simulink model "Time_10div"  (R2018a)
settings: Solver=VariableStepAuto  StartTime=0.0  StopTime=40  RelTol=1e-3
libraries: simulink_extras x8
settings Model: Creator=Liuinuy  LastModifiedBy=Liuinuy
settings OptimizationCC: BooleanDataType=off

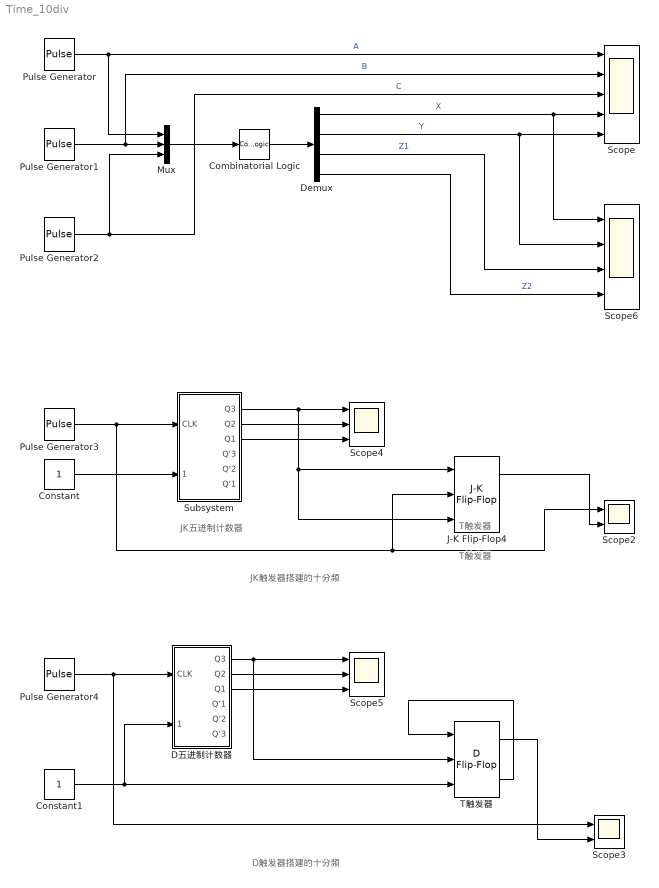
== system Time_10div ==
  note: T触发器
  note: JK触发器搭建的十分频
  note: D触发器搭建的十分频
  note: JK五进制计数器
  note: T触发器
  Combinatorial Logic : CombinatorialLogic  TruthTable=[1 1 1 1;1 0 1 0;1 0 1 0;1 0 1 0;1 0 1 0;1 0 1 0;1 0 1 0;0 1 1 0]
  Constant : Constant  OutDataTypeStr=boolean
  Constant1 : Constant  OutDataTypeStr=boolean
  Demux : Demux
  D五进制计数器 : Subsystem
  J-K Flip-Flop4 : simulink_extras/Flip Flops/J-K Flip-Flop  initial_condition=0
      settings: SourceProductName=Simulink
  Mux : Mux  Inputs=3
  Pulse Generator : DiscretePulseGenerator  Period=8  PulseWidth=4  PhaseDelay=4
  Pulse Generator1 : DiscretePulseGenerator  Period=4  PulseWidth=2  PhaseDelay=2
  Pulse Generator2 : DiscretePulseGenerator  PhaseDelay=1
  Pulse Generator3 : DiscretePulseGenerator
  Pulse Generator4 : DiscretePulseGenerator
  Scope : Scope  NumInputPorts=5
  Scope2 : Scope  NumInputPorts=2
  Scope3 : Scope  NumInputPorts=2
  Scope4 : Scope  NumInputPorts=3
  Scope5 : Scope  NumInputPorts=3
  Scope6 : Scope  NumInputPorts=4
  Subsystem : Subsystem
  T触发器 : simulink_extras/Flip Flops/D Flip-Flop
      settings: SourceProductName=Simulink
  wires:
  Pulse Generator/1 -> Mux/1, Scope/1  "A"
  Pulse Generator1/1 -> Scope/2, Mux/2  "B"
  Pulse Generator2/1 -> Mux/3, Scope/3  "C"
  Mux/1 -> Combinatorial Logic/1
  Combinatorial Logic/1 -> Demux/1
  Demux/1 -> Scope6/1, Scope/4  "X"
  Demux/2 -> Scope6/2, Scope/5  "Y"
  Demux/3 -> Scope6/3  "Z1"
  Demux/4 -> Scope6/4  "Z2"
  J-K Flip-Flop4/1 -> Scope2/2
  Pulse Generator4/1 -> Scope3/1, D五进制计数器/1(CLK)
  Constant1/1 -> D五进制计数器/2(1), T触发器/3
  T触发器/2 -> T触发器/1
  T触发器/1 -> Scope3/2
  Pulse Generator3/1 -> Subsystem/1(CLK), Scope2/1, J-K Flip-Flop4/2
  Subsystem/1(Q3) -> J-K Flip-Flop4/3, J-K Flip-Flop4/1, Scope4/1
  Constant/1 -> Subsystem/2(1)
  D五进制计数器/1(Q3) -> T触发器/2, Scope5/1
  D五进制计数器/3(Q1) -> Scope5/3
  D五进制计数器/2(Q2) -> Scope5/2
  Subsystem/2(Q2) -> Scope4/2
  Subsystem/3(Q1) -> Scope4/3

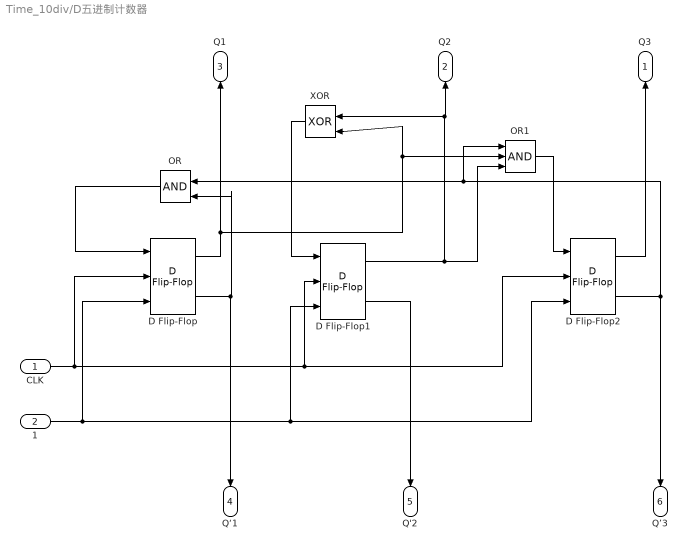
== system Time_10div/D五进制计数器 ==
  CLK : Inport
  1 : Inport  Port=2
  D Flip-Flop : simulink_extras/Flip Flops/D Flip-Flop
      settings: SourceProductName=Simulink
  D Flip-Flop1 : simulink_extras/Flip Flops/D Flip-Flop
      settings: SourceProductName=Simulink
  D Flip-Flop2 : simulink_extras/Flip Flops/D Flip-Flop
      settings: SourceProductName=Simulink
  OR : Logic  IconShape=distinctive  AllPortsSameDT=off  OutDataTypeStr=boolean
  OR1 : Logic  Inputs=3  IconShape=distinctive  AllPortsSameDT=off  OutDataTypeStr=boolean
  XOR : Logic  Operator=XOR  IconShape=distinctive  AllPortsSameDT=off  OutDataTypeStr=boolean
  Q3 : Outport
  Q2 : Outport  Port=2
  Q1 : Outport  Port=3
  Q‘1 : Outport  Port=4
  Q'2 : Outport  Port=5
  Q’3 : Outport  Port=6
  wires:
  D Flip-Flop/1 -> Q1/1, OR1/2, XOR/2
  OR/1 -> D Flip-Flop/1
  D Flip-Flop2/2 -> Q’3/1, OR1/1, OR/1
  OR1/1 -> D Flip-Flop2/1
  D Flip-Flop1/1 -> Q2/1, XOR/1, OR1/3
  CLK/1 -> D Flip-Flop/2, D Flip-Flop2/2, D Flip-Flop1/2
  XOR/1 -> D Flip-Flop1/1
  D Flip-Flop2/1 -> Q3/1
  D Flip-Flop/2 -> Q‘1/1, OR/2
  1/1 -> D Flip-Flop2/3, D Flip-Flop1/3, D Flip-Flop/3
  D Flip-Flop1/2 -> Q'2/1

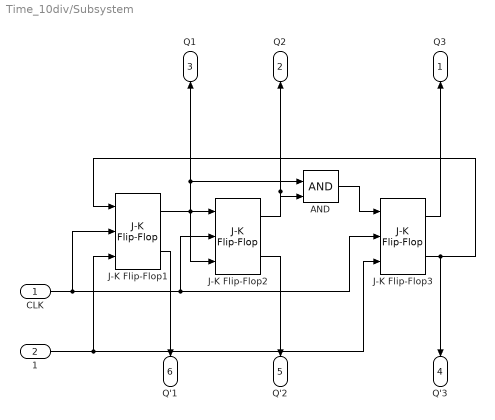
== system Time_10div/Subsystem ==
  CLK : Inport
  1 : Inport  Port=2
  AND : Logic  IconShape=distinctive  AllPortsSameDT=off  OutDataTypeStr=boolean
  J-K Flip-Flop1 : simulink_extras/Flip Flops/J-K Flip-Flop  initial_condition=0
      settings: SourceProductName=Simulink
  J-K Flip-Flop2 : simulink_extras/Flip Flops/J-K Flip-Flop  initial_condition=0
      settings: SourceProductName=Simulink
  J-K Flip-Flop3 : simulink_extras/Flip Flops/J-K Flip-Flop  initial_condition=0
      settings: SourceProductName=Simulink
  Q3 : Outport
  Q2 : Outport  Port=2
  Q1 : Outport  Port=3
  Q'3 : Outport  Port=4
  Q'2 : Outport  Port=5
  Q'1 : Outport  Port=6
  wires:
  CLK/1 -> J-K Flip-Flop3/2, J-K Flip-Flop2/2, J-K Flip-Flop1/2
  J-K Flip-Flop2/1 -> Q2/1, AND/2
  1/1 -> J-K Flip-Flop3/3, J-K Flip-Flop1/3
  J-K Flip-Flop3/2 -> Q'3/1, J-K Flip-Flop1/1
  AND/1 -> J-K Flip-Flop3/1
  J-K Flip-Flop1/1 -> J-K Flip-Flop2/1, J-K Flip-Flop2/3, AND/1, Q1/1
  J-K Flip-Flop3/1 -> Q3/1
  J-K Flip-Flop1/2 -> Q'1/1
  J-K Flip-Flop2/2 -> Q'2/1
